simulink subsystem "EvPowertrainController2EM_r3"  (R2023a)
settings: Solver=VariableStepAuto  StartTime=0.0  StopTime=10.0  RelTol=1e-3
undefined symbols (not defined in the file): CtrlVcuAccelPdlBpts, CtrlVcuBattPnlty, CtrlVcuEMPnlty, CtrlVcuEMTrqSplitGrid, CtrlVcuEvChrgLmtBpt, CtrlVcuEvRegenBrkCutOff, CtrlVcuEvRegenBrkSpdBpt, CtrlVcuEvSocBpt, CtrlVcuFallRate, CtrlVcuMaxAccelG, CtrlVcuMaxDecelG, CtrlVcuPwrRatePnlty, CtrlVcuRiseRate, CtrlVcuRoadMuEst, CtrlVcuSftyFctr, CtrlVcuTracPwrErrPnlty, CtrlVcuTrqVecBrkThresh, CtrlVcuTrqVecMinTrq, CtrlVcuTrqVecPGain, CtrlVcuTrqVecSteerThresh, CtrlVcuTrqVecVelThresh, DriverMode, eff, EnvGrvty, PlntBrkActrBoreFrnt, PlntBrkFrntBias, PlntBrkKinFricCffFrnt, PlntBrkNumPadsFrnt, PlntBrkPadMeanRadiusFrnt, PlntBrkPrsFctr, PlntBrkRearBias, PlntDiffrntl2Eff, PlntDiffrntl2Ratio, PlntDiffrntlEff, PlntDiffrntlRatio, PlntEM1EffTbl, PlntEM1Spd, PlntEM1Trq, PlntEM1TrqEff, PlntEM2EffTbl, PlntEM2Spd, PlntEM2Trq, PlntEM2TrqEff, PlntEM3EffTbl, PlntEM3Spd, PlntEM3Trq, PlntEM3TrqEff, PlntEMWhlGearEffFL, PlntEMWhlGearEffRL, PlntEMWhlGearRatioFL, PlntEMWhlGearRatioRL, PlntTransEffSpdBpt, PlntTransEffTbl, PlntTransEffTempBpt, PlntTransEffTrqBpt, PlntTransGearNumVect, PlntTransGearRatioVect, PlntVehCGHgtAxl, PlntVehDstCGFrntAxl, PlntVehDstCGRearAxl ... (+6)
libraries: simulink x19, autolibutils x2, slpidlib x2
(part 3 of 5)

== system EvPowertrainController2EM_r3/Energy Management/Convert Whl to EMTrq Vector/4EM/Gear Eta ==
  note: Pwr >= 0, v = 1
      | Pwr < 0, v= -1
  SpdIn : Inport
  TrqIn : Inport  Port=2
  Constant : Constant  Value=PlntEMWhlGearEffFL
  Constant1 : Constant  SampleTime=-1
  Constant2 : Constant  Value=-1  SampleTime=-1
  Math Function1 : Math  Operator=pow  SignedPower=on  OutputSignalType=real
  Product1 : Product
  Switch2 : Switch  SaturateOnIntegerOverflow=off  InputSameDT=off
  eta : Outport  VectorParamsAs1DForOutWhenUnconnected=off
  wires:
  SpdIn/1 -> Product1/2
  Constant/1 -> Math Function1/1
  Constant2/1 -> Switch2/3
  Constant1/1 -> Switch2/1
  Product1/1 -> Switch2/2
  Switch2/1 -> Math Function1/2
  Math Function1/1 -> eta/1
  TrqIn/1 -> Product1/1

== system EvPowertrainController2EM_r3/Energy Management/Convert Whl to EMTrq Vector/4EM/Gear Eta1 ==
  note: Pwr >= 0, v = 1
      | Pwr < 0, v= -1
  SpdIn : Inport
  TrqIn : Inport  Port=2
  Constant : Constant  Value=PlntEMWhlGearEffRL
  Constant1 : Constant  SampleTime=-1
  Constant2 : Constant  Value=-1  SampleTime=-1
  Math Function1 : Math  Operator=pow  SignedPower=on  OutputSignalType=real
  Product1 : Product
  Switch2 : Switch  SaturateOnIntegerOverflow=off  InputSameDT=off
  eta : Outport  VectorParamsAs1DForOutWhenUnconnected=off
  wires:
  TrqIn/1 -> Product1/1
  Math Function1/1 -> eta/1
  Switch2/1 -> Math Function1/2
  Product1/1 -> Switch2/2
  Constant1/1 -> Switch2/1
  Constant2/1 -> Switch2/3
  Constant/1 -> Math Function1/1
  SpdIn/1 -> Product1/2

== system EvPowertrainController2EM_r3/Energy Management/Powertrain Constraints /Battery Constraint/Electrical Current ==
  BattV : Inport
  EMPwrElecVec : Inport  Port=2
  DC-DC Eta : Subsystem  Variant=on  VariantControlMode=label  VariantControl=Variant1  LabelModeActiveChoice=0
  Divide : Product  Inputs=*/
  Saturation : Saturate  UpperLimit=Inf  LowerLimit=0.0001
  BatteryAmp : Outport  VectorParamsAs1DForOutWhenUnconnected=off
  wires:
  Saturation/1 -> Divide/2
  BattV/1 -> Saturation/1
  Divide/1 -> BatteryAmp/1
  EMPwrElecVec/1 -> DC-DC Eta/1(In)
  DC-DC Eta/1(Out) -> Divide/1

== system EvPowertrainController2EM_r3/Energy Management/Powertrain Constraints /Battery Constraint/Power Limit Calculations ==
  note: Use Current Limits from BMS to calculate
      | discharge and charge power limits
  BattPwrDisChrgLmt : Inport
  "BattPwrChrgLmt " : Inport  Port=2
  BattV_in : Inport  Port=3
  Data Type Conversion : DataTypeConversion  SaturateOnIntegerOverflow=off  RndMeth=Floor
  Data Type Conversion1 : DataTypeConversion  SaturateOnIntegerOverflow=off  RndMeth=Floor
  Divide : Product  Inputs=*/
  Divide1 : Product  Inputs=/*
  div0protect - poly : autolibutils/div0protect - poly  thresh=.01  ZeroCross=off  ZeroCross1=on  aMode=aMode
  div0protect - poly1 : autolibutils/div0protect - poly  thresh=.01  ZeroCross=off  ZeroCross1=on  aMode=aMode
  BattCurrDischrgLmt : Outport  VectorParamsAs1DForOutWhenUnconnected=off
  BattCurrChrgLmt : Outport  Port=2  VectorParamsAs1DForOutWhenUnconnected=off
  BattPwrDischrgLmt : Outport  Port=3  VectorParamsAs1DForOutWhenUnconnected=off
  BattPwrChrgLmt : Outport  Port=4  VectorParamsAs1DForOutWhenUnconnected=off
  wires:
  div0protect - poly1/1 -> Divide/2
  div0protect - poly/1 -> Divide1/1
  Divide1/1 -> BattCurrChrgLmt/1
  BattV_in/1 -> div0protect - poly1/1, div0protect - poly/1
  Divide/1 -> BattCurrDischrgLmt/1
  Data Type Conversion1/1 -> BattPwrDischrgLmt/1
  Data Type Conversion/1 -> BattPwrChrgLmt/1
  BattPwrDisChrgLmt/1 -> Data Type Conversion1/1, Divide/1
  "BattPwrChrgLmt "/1 -> Data Type Conversion/1, Divide1/2

== system EvPowertrainController2EM_r3/Energy Management/Powertrain Constraints /EM Constraint Front/Maximum Torque ==
  note: Don't allow negative MotTrq when
      | WhlTrqCmd is >= 0
  WhlTrqCmd : Inport
  WhlEMTrqSplitVecFrnt : Inport  Port=2
  WhlTrqMaxVec : Inport  Port=3
  Compare To Zero : simulink/Logic and Bit Operations/Compare To Zero  relop=<  OutDataTypeStr=boolean
  Compare To Zero1 : simulink/Logic and Bit Operations/Compare To Zero  relop=>=  OutDataTypeStr=boolean
  Gain : Gain  Gain=-1
  Logical Operator : Logic  Operator=OR  Inputs=3  AllPortsSameDT=off  OutDataTypeStr=boolean
  Logical Operator1 : Logic  AllPortsSameDT=off  OutDataTypeStr=boolean
  Relational Operator : RelationalOperator  Operator=<  OutDataTypeStr=boolean  RndMeth=Simplest  InputSameDT=off
  Relational Operator1 : RelationalOperator  Operator=<  OutDataTypeStr=boolean  RndMeth=Simplest  InputSameDT=off
  Saturation Dynamic : simulink/Discontinuities/Saturation Dynamic  OutMin=[]  OutMax=[]  OutDataTypeStr=Inherit: Same as second input  OutDataType=fixdt(1, 16)  OutScaling=2^-10  DoSatur=off
  WhlEMTrqSatVec : Outport  VectorParamsAs1DForOutWhenUnconnected=off
  InfeasibleEMVec : Outport  Port=2  VectorParamsAs1DForOutWhenUnconnected=off
  wires:
  WhlTrqMaxVec/1 -> Saturation Dynamic/1, Relational Operator/1, Gain/1
  Logical Operator/1 -> InfeasibleEMVec/1
  Relational Operator1/1 -> Logical Operator/2
  Relational Operator/1 -> Logical Operator/1
  Saturation Dynamic/1 -> WhlEMTrqSatVec/1
  Gain/1 -> Saturation Dynamic/3, Relational Operator1/2
  WhlTrqCmd/1 -> Compare To Zero1/1
  Compare To Zero/1 -> Logical Operator1/1
  WhlEMTrqSplitVecFrnt/1 -> Compare To Zero/1, Saturation Dynamic/2, Relational Operator1/1, Relational Operator/2
  Compare To Zero1/1 -> Logical Operator1/2
  Logical Operator1/1 -> Logical Operator/3

== system EvPowertrainController2EM_r3/Energy Management/Powertrain Constraints /EM Constraint Front/Tabular Power Loss Data ==
  EMAvgSpdVec : Inport
  WhlEMTrqSatVec : Inport  Port=2
  2EM or 3EM Dual Rear : Subsystem  VariantControl=2EM or 3EM Dual Rear
  3EM Dual Front or 4EM : Subsystem  VariantControl=3EM Dual Front or 4EM
  EMPwrElecVec : Outport

== system EvPowertrainController2EM_r3/Energy Management/Powertrain Constraints /EM Constraint Front/Wheel Torque Saturation for Max g Rates ==
  WhlTrqCmd : Inport
  Tqin : Inport  Port=2
  Constant : Constant  Value=0  SampleTime=-1
  Road mu : Gain  Gain=CtrlVcuRoadMuEst
  Road mu1 : Gain  Gain=CtrlVcuRoadMuEst
  Safety Factor : Gain  Gain=CtrlVcuSftyFctr
  Safety Factor1 : Gain  Gain=CtrlVcuSftyFctr
  Saturation Dynamic3 : simulink/Discontinuities/Saturation Dynamic  OutMin=[]  OutMax=[]  OutDataTypeStr=Inherit: Same as second input  OutDataType=fixdt(1, 16)  OutScaling=2^-10  DoSatur=off
  Selector4 : Selector  InputPortWidth=2  IndexOptions=Index vector (dialog)  Indices=1  OutputSizes=1
  Selector6 : Selector  InputPortWidth=2  IndexOptions=Index vector (dialog)  Indices=1  OutputSizes=1
  Switch : Switch  Criteria=u2 > Threshold  SaturateOnIntegerOverflow=off  InputSameDT=off
  Switch1 : Switch  Criteria=u2 > Threshold  SaturateOnIntegerOverflow=off  InputSameDT=off
  Wheel Torque Limit at Max g Rates : Subsystem
  tqOut : Outport
  wires:
  WhlTrqCmd/1 -> Switch1/2, Switch/2
  Constant/1 -> Switch1/1, Switch/3
  Switch1/1 -> Saturation Dynamic3/3
  Switch/1 -> Saturation Dynamic3/1
  Safety Factor1/1 -> Switch1/3
  Safety Factor/1 -> Switch/1
  Road mu1/1 -> Safety Factor1/1
  Road mu/1 -> Safety Factor/1
  Wheel Torque Limit at Max g Rates/2(WhlTrqLmt_Brk) -> Selector6/1
  Saturation Dynamic3/1 -> tqOut/1
  Tqin/1 -> Saturation Dynamic3/2
  Selector4/1 -> Road mu/1
  Wheel Torque Limit at Max g Rates/1(WhlTrqLmt_Accel) -> Selector4/1
  Selector6/1 -> Road mu1/1

== system EvPowertrainController2EM_r3/Energy Management/Powertrain Constraints /EM Constraint Rear/Maximum Torque ==
  note: Don't allow negative MotTrq when
      | WhlTrqCmd is >= 0
  WhlTrqCmd : Inport
  WhlEMTrqSplitVecRear : Inport  Port=2
  WhlTrqMaxVec : Inport  Port=3
  Compare To Zero : simulink/Logic and Bit Operations/Compare To Zero  relop=<  OutDataTypeStr=boolean
  Compare To Zero1 : simulink/Logic and Bit Operations/Compare To Zero  relop=>=  OutDataTypeStr=boolean
  Gain : Gain  Gain=-1
  Logical Operator : Logic  Operator=OR  Inputs=3  AllPortsSameDT=off  OutDataTypeStr=boolean
  Logical Operator1 : Logic  AllPortsSameDT=off  OutDataTypeStr=boolean
  Relational Operator : RelationalOperator  Operator=<  OutDataTypeStr=boolean  RndMeth=Simplest  InputSameDT=off
  Relational Operator1 : RelationalOperator  Operator=<  OutDataTypeStr=boolean  RndMeth=Simplest  InputSameDT=off
  Saturation Dynamic : simulink/Discontinuities/Saturation Dynamic  OutMin=[]  OutMax=[]  OutDataTypeStr=Inherit: Same as second input  OutDataType=fixdt(1, 16)  OutScaling=2^-10  DoSatur=off
  WhlEMTrqSatVec : Outport  VectorParamsAs1DForOutWhenUnconnected=off
  InfeasibleEMVec : Outport  Port=2  VectorParamsAs1DForOutWhenUnconnected=off
  wires:
  Logical Operator1/1 -> Logical Operator/3
  Compare To Zero1/1 -> Logical Operator1/2
  WhlEMTrqSplitVecRear/1 -> Relational Operator/2, Relational Operator1/1, Saturation Dynamic/2, Compare To Zero/1
  Compare To Zero/1 -> Logical Operator1/1
  WhlTrqCmd/1 -> Compare To Zero1/1
  Gain/1 -> Relational Operator1/2, Saturation Dynamic/3
  Saturation Dynamic/1 -> WhlEMTrqSatVec/1
  Relational Operator/1 -> Logical Operator/1
  Relational Operator1/1 -> Logical Operator/2
  Logical Operator/1 -> InfeasibleEMVec/1
  WhlTrqMaxVec/1 -> Gain/1, Relational Operator/1, Saturation Dynamic/1

== system EvPowertrainController2EM_r3/Energy Management/Powertrain Constraints /EM Constraint Rear/Tabular Power Loss Data ==
  EMAvgSpdVec : Inport
  WhlEMTrqSatVec : Inport  Port=2
  2EM : Subsystem  VariantControl=2EM
  3EM Dual Front : Subsystem  VariantControl=3EM Dual Front
  3EM Dual Rear or 4EM : Subsystem  VariantControl=3EM Dual Rear or 4EM
  EMPwrElecVec : Outport

== system EvPowertrainController2EM_r3/Energy Management/Powertrain Constraints /EM Constraint Rear/Wheel Torque Saturation for Max g Rates ==
  WhlTrqCmd : Inport
  Tqin : Inport  Port=2
  Constant : Constant  Value=0  SampleTime=-1
  Road mu : Gain  Gain=CtrlVcuRoadMuEst
  Road mu1 : Gain  Gain=CtrlVcuRoadMuEst
  Safety Factor : Gain  Gain=CtrlVcuSftyFctr
  Safety Factor1 : Gain  Gain=CtrlVcuSftyFctr
  Saturation Dynamic3 : simulink/Discontinuities/Saturation Dynamic  OutMin=[]  OutMax=[]  OutDataTypeStr=Inherit: Same as second input  OutDataType=fixdt(1, 16)  OutScaling=2^-10  DoSatur=off
  Selector4 : Selector  InputPortWidth=2  IndexOptions=Index vector (dialog)  Indices=2  OutputSizes=1
  Selector6 : Selector  InputPortWidth=2  IndexOptions=Index vector (dialog)  Indices=2  OutputSizes=1
  Switch : Switch  Criteria=u2 > Threshold  SaturateOnIntegerOverflow=off  InputSameDT=off
  Switch1 : Switch  Criteria=u2 > Threshold  SaturateOnIntegerOverflow=off  InputSameDT=off
  Wheel Torque Limit at Max g Rates : Subsystem
  tqOut : Outport
  wires:
  WhlTrqCmd/1 -> Switch1/2, Switch/2
  Constant/1 -> Switch1/1, Switch/3
  Switch1/1 -> Saturation Dynamic3/3
  Switch/1 -> Saturation Dynamic3/1
  Safety Factor1/1 -> Switch1/3
  Safety Factor/1 -> Switch/1
  Road mu1/1 -> Safety Factor1/1
  Road mu/1 -> Safety Factor/1
  Wheel Torque Limit at Max g Rates/2(WhlTrqLmt_Brk) -> Selector6/1
  Saturation Dynamic3/1 -> tqOut/1
  Tqin/1 -> Saturation Dynamic3/2
  Selector4/1 -> Road mu/1
  Wheel Torque Limit at Max g Rates/1(WhlTrqLmt_Accel) -> Selector4/1
  Selector6/1 -> Road mu1/1

== system EvPowertrainController2EM_r3/Energy Management/Powertrain Constraints /Wheel Torque Vector Logic/Regen ==
  note: 2. If #1 is false:
      |
      | Rear Torque = Rear Torque Split Vector
  note: 2. If #1 is true:
      |
      | Rear Torque = WhlTrqCmd - WhlTrqSplitVecFront (Saturated)
  note: Check if WhlTrqCmd >= WhlTrqSplitVecFront
  note: Regen Torques are Negative
  note: Ensures rear torques never greater than
      | front torques during braking
  WhlTrqCmd : Inport
  WhlEMTrqSatVecFrnt : Inport  Port=2
  WhlEMTrqSplitVecFrnt : Inport  Port=3
  WhlEMTrqSplitVecRear : Inport  Port=4
  Action Port : ActionPort
  Add3 : Sum  Inputs=+-
  Constant1 : Constant  Value=0  SampleTime=-1
  Relational Operator : RelationalOperator  OutDataTypeStr=boolean  RndMeth=Simplest  InputSameDT=off
  Saturation Dynamic : simulink/Discontinuities/Saturation Dynamic  OutMin=[]  OutMax=[]  OutDataTypeStr=Inherit: Same as second input  OutDataType=fixdt(1, 16)  OutScaling=2^-10  DoSatur=off
  Switch1 : Switch  Criteria=u2 > Threshold  SaturateOnIntegerOverflow=off  InputSameDT=off
  WhlEMTrqSplitVecFrnt1 : Outport
  WhlEMTrqSplitVecRear1 : Outport  Port=2
  wires:
  WhlEMTrqSplitVecRear/1 -> Switch1/3
  Constant1/1 -> Saturation Dynamic/1
  Switch1/1 -> Saturation Dynamic/2
  Relational Operator/1 -> Switch1/2
  Add3/1 -> Switch1/1
  WhlEMTrqSatVecFrnt/1 -> Add3/2
  WhlTrqCmd/1 -> Relational Operator/1, Add3/1
  Saturation Dynamic/1 -> WhlEMTrqSplitVecRear1/1  "WhlEMTrqSplitVecRear"
  WhlEMTrqSplitVecFrnt/1 -> Relational Operator/2, WhlEMTrqSplitVecFrnt1/1, Saturation Dynamic/3  "WhlEMTrqSplitVecFrnt"

== system EvPowertrainController2EM_r3/Energy Management/Powertrain Constraints /Wheel Torque Vector Logic/Traction ==
  note: 2. If #1 is false:
      |
      | Front Torque = Front Torque Split Vector
  note: Check if WhlTrqCmd <= WhlTrqSplitVecRear
  note: 2. If #1 is true:
      |
      | Front Torque = WhlTrqCmd - WhlTrqSplitVecRear (Saturated)
  WhlTrqCmd : Inport
  WhlEMTrqSatVecRear : Inport  Port=2
  WhlEMTrqSplitVecFrnt : Inport  Port=3
  WhlEMTrqSplitVecRear : Inport  Port=4
  Action Port : ActionPort
  Add3 : Sum  Inputs=+-
  Relational Operator : RelationalOperator  Operator=<=  OutDataTypeStr=boolean  RndMeth=Simplest  InputSameDT=off
  Switch1 : Switch  Criteria=u2 > Threshold  SaturateOnIntegerOverflow=off  InputSameDT=off
  WhlEMTrqSplitVecFrnt1 : Outport
  WhlEMTrqSplitVecRear1 : Outport  Port=2
  wires:
  WhlEMTrqSplitVecRear/1 -> Relational Operator/2, WhlEMTrqSplitVecRear1/1  "WhlEMTrqSplitVecRear"
  Relational Operator/1 -> Switch1/2
  WhlEMTrqSplitVecFrnt/1 -> Switch1/3
  Switch1/1 -> WhlEMTrqSplitVecFrnt1/1  "WhlEMTrqSplitVecFrnt"
  WhlTrqCmd/1 -> Add3/1, Relational Operator/1
  WhlEMTrqSatVecRear/1 -> Add3/2
  Add3/1 -> Switch1/1

== system EvPowertrainController2EM_r3/Torque Vectoring/3EM/Create EMTrq Vector/3EMDualFront ==
  EMTrqSplit : Inport
  EMTrqCmd : Inport  Port=2
  Selector : Selector  InputPortWidth=3  IndexOptions=Index vector (dialog)  Indices=[3]  OutputSizes=1
  Vector Concatenate : Concatenate
  EMTrqCmdFinal : Outport
  wires:
  EMTrqSplit/1 -> Vector Concatenate/1
  Vector Concatenate/1 -> EMTrqCmdFinal/1
  EMTrqCmd/1 -> Selector/1
  Selector/1 -> Vector Concatenate/2

== system EvPowertrainController2EM_r3/Torque Vectoring/3EM/Create EMTrq Vector/3EMDualRear ==
  EMTrqSplit : Inport
  EMTrqCmd : Inport  Port=2
  Selector : Selector  InputPortWidth=3  IndexOptions=Index vector (dialog)  Indices=[1]  OutputSizes=1
  Vector Concatenate : Concatenate
  EMTrqCmdFinal : Outport
  wires:
  EMTrqCmd/1 -> Selector/1
  Vector Concatenate/1 -> EMTrqCmdFinal/1
  EMTrqSplit/1 -> Vector Concatenate/2
  Selector/1 -> Vector Concatenate/1

== system EvPowertrainController2EM_r3/Torque Vectoring/3EM/EMTrq/3EMDualFront ==
  EMSpd : Inport
  EMTrqCmd : Inport  Port=2
  1-D Lookup Table : Lookup_n-D  NumberOfTableDimensions=1  BreakpointsForDimension1=PlntEM1Spd  Table=PlntEM1Trq  ExtrapMethod=Clip  UseLastTableValue=on  InternalRulePriority=Speed  RndMeth=Simplest
  3EMDualFront : Subsystem  VariantControl=3EMDualFront
  Abs1 : Abs  SaturateOnIntegerOverflow=off
  Abs2 : Abs  SaturateOnIntegerOverflow=off
  Selector : Selector  InputPortWidth=3  IndexOptions=Index vector (dialog)  Indices=[1]  OutputSizes=1
  Selector1 : Selector  InputPortWidth=3  IndexOptions=Index vector (dialog)  Indices=[2]  OutputSizes=1
  EMTrqMax : Outport
  EMTrqL : Outport  Port=2
  EMTrqR : Outport  Port=3
  wires:
  Abs2/1 -> EMTrqMax/1
  Abs1/1 -> 1-D Lookup Table/1
  EMSpd/1 -> 3EMDualFront/1(EMSpd)
  1-D Lookup Table/1 -> Abs2/1
  3EMDualFront/1(EMSpdAvg) -> Abs1/1
  EMTrqCmd/1 -> Selector1/1, Selector/1
  Selector/1 -> EMTrqL/1
  Selector1/1 -> EMTrqR/1

== system EvPowertrainController2EM_r3/Torque Vectoring/3EM/EMTrq/3EMDualRear ==
  EMSpd : Inport
  EMTrqCmd : Inport  Port=2
  1-D Lookup Table : Lookup_n-D  NumberOfTableDimensions=1  BreakpointsForDimension1=PlntEM3Spd  Table=PlntEM3Trq  ExtrapMethod=Clip  UseLastTableValue=on  InternalRulePriority=Speed  RndMeth=Simplest
  3EMDualRear : Subsystem  VariantControl=3EMDualRear
  Abs1 : Abs  SaturateOnIntegerOverflow=off
  Abs2 : Abs  SaturateOnIntegerOverflow=off
  Selector : Selector  InputPortWidth=3  IndexOptions=Index vector (dialog)  Indices=[2]  OutputSizes=1
  Selector1 : Selector  InputPortWidth=3  IndexOptions=Index vector (dialog)  Indices=[3]  OutputSizes=1
  EMTrqMax : Outport
  EMTrqL : Outport  Port=2
  EMTrqR : Outport  Port=3
  wires:
  Abs2/1 -> EMTrqMax/1
  3EMDualRear/1(EMSpdAvg) -> Abs1/1
  1-D Lookup Table/1 -> Abs2/1
  EMSpd/1 -> 3EMDualRear/1(EMSpd)
  Abs1/1 -> 1-D Lookup Table/1
  Selector1/1 -> EMTrqR/1
  Selector/1 -> EMTrqL/1
  EMTrqCmd/1 -> Selector1/1, Selector/1

== system EvPowertrainController2EM_r3/Torque Vectoring/4EM/EMTrq/Dual Front ==
  EMSpd : Inport
  EMTrqCmd : Inport  Port=2
  1-D Lookup Table : Lookup_n-D  NumberOfTableDimensions=1  BreakpointsForDimension1=PlntEM1Spd  Table=PlntEM1Trq  ExtrapMethod=Clip  UseLastTableValue=on  InternalRulePriority=Speed  RndMeth=Simplest
  3EMDualFrnt : Subsystem  VariantControl=3EMDualFront
  Abs1 : Abs  SaturateOnIntegerOverflow=off
  Abs2 : Abs  SaturateOnIntegerOverflow=off
  Selector : Selector  InputPortWidth=4  IndexOptions=Index vector (dialog)  Indices=[1]  OutputSizes=1
  Selector1 : Selector  InputPortWidth=4  IndexOptions=Index vector (dialog)  Indices=[2]  OutputSizes=1
  EMTrqMaxFrnt : Outport
  EMTrqFL : Outport  Port=2
  EMTrqFR : Outport  Port=3
  wires:
  Abs2/1 -> EMTrqMaxFrnt/1
  Selector1/1 -> EMTrqFR/1
  Selector/1 -> EMTrqFL/1
  EMTrqCmd/1 -> Selector/1, Selector1/1
  3EMDualFrnt/1(EMSpdAvg) -> Abs1/1
  1-D Lookup Table/1 -> Abs2/1
  EMSpd/1 -> 3EMDualFrnt/1(EMSpd)
  Abs1/1 -> 1-D Lookup Table/1

== system EvPowertrainController2EM_r3/Torque Vectoring/4EM/EMTrq/Dual Rear ==
  EMSpd : Inport
  EMTrqCmd : Inport  Port=2
  1-D Lookup Table : Lookup_n-D  NumberOfTableDimensions=1  BreakpointsForDimension1=PlntEM3Spd  Table=PlntEM3Trq  ExtrapMethod=Clip  UseLastTableValue=on  InternalRulePriority=Speed  RndMeth=Simplest
  3EMDualRear : Subsystem  VariantControl=3EMDualRear
  Abs1 : Abs  SaturateOnIntegerOverflow=off
  Abs2 : Abs  SaturateOnIntegerOverflow=off
  Selector : Selector  InputPortWidth=4  IndexOptions=Index vector (dialog)  Indices=[3]  OutputSizes=1
  Selector1 : Selector  InputPortWidth=4  IndexOptions=Index vector (dialog)  Indices=[4]  OutputSizes=1
  EMTrqMaxRear : Outport
  EMTrqRL : Outport  Port=2
  EMTrqRR : Outport  Port=3
  wires:
  Abs2/1 -> EMTrqMaxRear/1
  EMTrqCmd/1 -> Selector/1, Selector1/1
  Selector/1 -> EMTrqRL/1
  Selector1/1 -> EMTrqRR/1
  Abs1/1 -> 1-D Lookup Table/1
  EMSpd/1 -> 3EMDualRear/1(EMSpd)
  1-D Lookup Table/1 -> Abs2/1
  3EMDualRear/1(EMSpdAvg) -> Abs1/1

== system EvPowertrainController2EM_r3/Accel Pedal to Traction Wheel Torque Request/EM2WhlTrq/2EM/EMTrq2WhlTrqFrnt/No Transmission ==
  EMTrqCmd : Inport
  EMSpd : Inport  Port=2
  Diff Eta : Subsystem
  Divide2 : Product  Inputs=**
  Gain3 : Gain  Gain=PlntDiffrntlRatio
  WhlMotTrq : Outport  VectorParamsAs1DForOutWhenUnconnected=off
  wires:
  Gain3/1 -> Divide2/2
  Divide2/1 -> WhlMotTrq/1
  EMSpd/1 -> Diff Eta/1(SpdIn)
  EMTrqCmd/1 -> Diff Eta/2(TrqIn), Gain3/1
  Diff Eta/1(eta) -> Divide2/1

== system EvPowertrainController2EM_r3/Accel Pedal to Traction Wheel Torque Request/EM2WhlTrq/2EM/EMTrq2WhlTrqFrnt/Transmission ==
  Gear : Inport
  EMTrqCmd : Inport  Port=2
  EMSpd : Inport  Port=3
  Diff Eta : Subsystem
  Divide : Product  Inputs=**
  Divide1 : Product  Inputs=**
  Divide2 : Product  Inputs=**
  Divide3 : Product  Inputs=*/
  Gain : Gain  Gain=PlntDiffrntlRatio
  Gear ratio look up : LookupNDDirect  NumberOfTableDimensions=1  Table=PlntTransGearRatioVect
  Trans Eta : Subsystem
  WhlMotTrq : Outport  VectorParamsAs1DForOutWhenUnconnected=off
  wires:
  EMSpd/1 -> Trans Eta/2(SpdIn), [Spd]
  EMTrqCmd/1 -> Trans Eta/1(TrqIn), Divide/2
  Divide3/1 -> Diff Eta/1(SpdIn)
  [Spd] -> Divide3/1
  Diff Eta/1(eta) -> Divide2/1
  Divide2/1 -> WhlMotTrq/1
  Divide1/1 -> Gain/1, Diff Eta/2(TrqIn)
  Trans Eta/1(eta) -> Divide1/1
  Gear/1 -> Gear ratio look up/1, Trans Eta/3(Gear)
  Divide/1 -> Divide1/2
  Gear ratio look up/1 -> Divide/1, Divide3/2
  Gain/1 -> Divide2/2

== system EvPowertrainController2EM_r3/Accel Pedal to Traction Wheel Torque Request/EM2WhlTrq/2EM/EMTrq2WhlTrqRear/No Transmission ==
  EMTrqCmd : Inport
  EMSpd : Inport  Port=2
  Diff Eta : Subsystem
  Divide2 : Product  Inputs=**
  Gain3 : Gain  Gain=PlntDiffrntl2Ratio
  WhlMotTrq : Outport  VectorParamsAs1DForOutWhenUnconnected=off
  wires:
  Gain3/1 -> Divide2/2
  Divide2/1 -> WhlMotTrq/1
  EMSpd/1 -> Diff Eta/1(SpdIn)
  EMTrqCmd/1 -> Diff Eta/2(TrqIn), Gain3/1
  Diff Eta/1(eta) -> Divide2/1

== system EvPowertrainController2EM_r3/Accel Pedal to Traction Wheel Torque Request/EM2WhlTrq/2EM/EMTrq2WhlTrqRear/Transmission ==
  Gear : Inport
  EMTrqCmd : Inport  Port=2
  EMSpd : Inport  Port=3
  Diff Eta : Subsystem
  Divide : Product  Inputs=**
  Divide1 : Product  Inputs=**
  Divide2 : Product  Inputs=**
  Divide3 : Product  Inputs=*/
  Gain : Gain  Gain=PlntDiffrntl2Ratio
  Gear ratio look up : LookupNDDirect  NumberOfTableDimensions=1  Table=PlntTransGearRatioVect
  Trans Eta : Subsystem
  WhlMotTrq : Outport  VectorParamsAs1DForOutWhenUnconnected=off
  wires:
  Gain/1 -> Divide2/2
  Gear ratio look up/1 -> Divide3/2, Divide/1
  Divide/1 -> Divide1/2
  Gear/1 -> Trans Eta/3(Gear), Gear ratio look up/1
  Trans Eta/1(eta) -> Divide1/1
  Divide1/1 -> Diff Eta/2(TrqIn), Gain/1
  Divide2/1 -> WhlMotTrq/1
  Diff Eta/1(eta) -> Divide2/1
  [Spd] -> Divide3/1
  Divide3/1 -> Diff Eta/1(SpdIn)
  EMTrqCmd/1 -> Divide/2, Trans Eta/1(TrqIn)
  EMSpd/1 -> [Spd], Trans Eta/2(SpdIn)

== system EvPowertrainController2EM_r3/Accel Pedal to Traction Wheel Torque Request/EM2WhlTrq/2EM/VehSpd2EMSpd/No Transmission ==
  VehSpd : Inport
  Gain1 : Gain  Gain=PlntDiffrntlRatio
  Gain2 : Gain  Gain=PlntDiffrntl2Ratio
  Gain3 : Gain  Gain=1 / PlntWhlLdRadius
  EMSpdFrntAxl : Outport  VectorParamsAs1DForOutWhenUnconnected=off
  EMSpdRearAxl : Outport  Port=2  VectorParamsAs1DForOutWhenUnconnected=off
  wires:
  Gain2/1 -> EMSpdRearAxl/1
  Gain3/1 -> Gain2/1, Gain1/1
  Gain1/1 -> EMSpdFrntAxl/1
  VehSpd/1 -> Gain3/1

== system EvPowertrainController2EM_r3/Accel Pedal to Traction Wheel Torque Request/EM2WhlTrq/2EM/VehSpd2EMSpd/Transmission ==
  Gear : Inport
  VehSpd : Inport  Port=2
  Divide1 : Product  Inputs=**
  Gain1 : Gain  Gain=PlntDiffrntlRatio
  Gain2 : Gain  Gain=PlntDiffrntl2Ratio
  Gain3 : Gain  Gain=1 / PlntWhlLdRadius
  Gear ratio look up : LookupNDDirect  NumberOfTableDimensions=1  Table=PlntTransGearRatioVect
  EMSpdFrntAxl : Outport  VectorParamsAs1DForOutWhenUnconnected=off
  EMSpdRearAxl : Outport  Port=2  VectorParamsAs1DForOutWhenUnconnected=off
  wires:
  Divide1/1 -> EMSpdRearAxl/1
  Gain2/1 -> Divide1/2
  Gear ratio look up/1 -> Divide1/1
  Gain1/1 -> EMSpdFrntAxl/1
  Gain3/1 -> Gain1/1, Gain2/1
  Gear/1 -> Gear ratio look up/1
  VehSpd/1 -> Gain3/1

== system EvPowertrainController2EM_r3/Accel Pedal to Traction Wheel Torque Request/EM2WhlTrq/3EM Dual Front/EMTrq2WhlTrqFrnt/No Transmission ==
  EMTrqCmd : Inport
  EMSpd : Inport  Port=2
  Divide2 : Product  Inputs=**
  Dual EMs : Gain  Gain=2
  Gain3 : Gain  Gain=PlntEMWhlGearRatioFL
  Gear Eta : Subsystem
  WhlMotTrq : Outport  VectorParamsAs1DForOutWhenUnconnected=off
  wires:
  Dual EMs/1 -> Gain3/1, Gear Eta/2(TrqIn)
  Gear Eta/1(eta) -> Divide2/1
  EMTrqCmd/1 -> Dual EMs/1
  EMSpd/1 -> Gear Eta/1(SpdIn)
  Divide2/1 -> WhlMotTrq/1
  Gain3/1 -> Divide2/2

== system EvPowertrainController2EM_r3/Accel Pedal to Traction Wheel Torque Request/EM2WhlTrq/3EM Dual Front/EMTrq2WhlTrqFrnt/Transmission ==
  Gear : Inport
  EMTrqCmd : Inport  Port=2
  EMSpd : Inport  Port=3
  Diff Eta : Subsystem
  Divide : Product  Inputs=**
  Divide1 : Product  Inputs=**
  Divide2 : Product  Inputs=**
  Divide3 : Product  Inputs=*/
  Gain : Gain  Gain=PlntDiffrntlRatio
  Gear ratio look up : LookupNDDirect  NumberOfTableDimensions=1  Table=PlntTransGearRatioVect
  Trans Eta : Subsystem
  WhlMotTrq : Outport  VectorParamsAs1DForOutWhenUnconnected=off
  wires:
  Gain/1 -> Divide2/2
  Gear ratio look up/1 -> Divide3/2, Divide/1
  Divide/1 -> Divide1/2
  Gear/1 -> Trans Eta/3(Gear), Gear ratio look up/1
  Trans Eta/1(eta) -> Divide1/1
  Divide1/1 -> Diff Eta/2(TrqIn), Gain/1
  Divide2/1 -> WhlMotTrq/1
  Diff Eta/1(eta) -> Divide2/1
  [Spd] -> Divide3/1
  Divide3/1 -> Diff Eta/1(SpdIn)
  EMTrqCmd/1 -> Divide/2, Trans Eta/1(TrqIn)
  EMSpd/1 -> [Spd], Trans Eta/2(SpdIn)

== system EvPowertrainController2EM_r3/Accel Pedal to Traction Wheel Torque Request/EM2WhlTrq/3EM Dual Front/EMTrq2WhlTrqRear/No Transmission ==
  EMTrqCmd : Inport
  EMSpd : Inport  Port=2
  Diff Eta : Subsystem
  Divide2 : Product  Inputs=**
  Gain3 : Gain  Gain=PlntDiffrntl2Ratio
  WhlMotTrq : Outport  VectorParamsAs1DForOutWhenUnconnected=off
  wires:
  Diff Eta/1(eta) -> Divide2/1
  EMTrqCmd/1 -> Gain3/1, Diff Eta/2(TrqIn)
  EMSpd/1 -> Diff Eta/1(SpdIn)
  Divide2/1 -> WhlMotTrq/1
  Gain3/1 -> Divide2/2

== system EvPowertrainController2EM_r3/Accel Pedal to Traction Wheel Torque Request/EM2WhlTrq/3EM Dual Front/EMTrq2WhlTrqRear/Transmission ==
  Gear : Inport
  EMTrqCmd : Inport  Port=2
  EMSpd : Inport  Port=3
  Diff Eta : Subsystem
  Divide : Product  Inputs=**
  Divide1 : Product  Inputs=**
  Divide2 : Product  Inputs=**
  Divide3 : Product  Inputs=*/
  Gain : Gain  Gain=PlntDiffrntl2Ratio
  Gear ratio look up : LookupNDDirect  NumberOfTableDimensions=1  Table=PlntTransGearRatioVect
  Trans Eta : Subsystem
  WhlMotTrq : Outport  VectorParamsAs1DForOutWhenUnconnected=off
  wires:
  EMSpd/1 -> Trans Eta/2(SpdIn), [Spd]
  EMTrqCmd/1 -> Trans Eta/1(TrqIn), Divide/2
  Divide3/1 -> Diff Eta/1(SpdIn)
  [Spd] -> Divide3/1
  Diff Eta/1(eta) -> Divide2/1
  Divide2/1 -> WhlMotTrq/1
  Divide1/1 -> Gain/1, Diff Eta/2(TrqIn)
  Trans Eta/1(eta) -> Divide1/1
  Gear/1 -> Gear ratio look up/1, Trans Eta/3(Gear)
  Divide/1 -> Divide1/2
  Gear ratio look up/1 -> Divide/1, Divide3/2
  Gain/1 -> Divide2/2

== system EvPowertrainController2EM_r3/Accel Pedal to Traction Wheel Torque Request/EM2WhlTrq/3EM Dual Front/VehSpd2EMSpd/No Transmission ==
  VehSpd : Inport
  Gain1 : Gain  Gain=PlntEMWhlGearRatioFL
  Gain2 : Gain  Gain=PlntDiffrntl2Ratio
  Gain3 : Gain  Gain=1 / PlntWhlLdRadius
  EMSpdFrntAxl : Outport  VectorParamsAs1DForOutWhenUnconnected=off
  EMSpdRearAxl : Outport  Port=2  VectorParamsAs1DForOutWhenUnconnected=off
  wires:
  VehSpd/1 -> Gain3/1
  Gain1/1 -> EMSpdFrntAxl/1
  Gain3/1 -> Gain1/1, Gain2/1
  Gain2/1 -> EMSpdRearAxl/1

== system EvPowertrainController2EM_r3/Accel Pedal to Traction Wheel Torque Request/EM2WhlTrq/3EM Dual Front/VehSpd2EMSpd/Transmission ==
  Gear : Inport
  VehSpd : Inport  Port=2
  Divide1 : Product  Inputs=**
  Gain1 : Gain  Gain=PlntDiffrntlRatio
  Gain2 : Gain  Gain=PlntDiffrntl2Ratio
  Gain3 : Gain  Gain=1 / PlntWhlLdRadius
  Gear ratio look up : LookupNDDirect  NumberOfTableDimensions=1  Table=PlntTransGearRatioVect
  EMSpdFrntAxl : Outport  VectorParamsAs1DForOutWhenUnconnected=off
  EMSpdRearAxl : Outport  Port=2  VectorParamsAs1DForOutWhenUnconnected=off
  wires:
  VehSpd/1 -> Gain3/1
  Gear/1 -> Gear ratio look up/1
  Gain3/1 -> Gain2/1, Gain1/1
  Gain1/1 -> EMSpdFrntAxl/1
  Gear ratio look up/1 -> Divide1/1
  Gain2/1 -> Divide1/2
  Divide1/1 -> EMSpdRearAxl/1

== system EvPowertrainController2EM_r3/Accel Pedal to Traction Wheel Torque Request/EM2WhlTrq/3EM Dual Rear/EMTrq2WhlTrqFrnt/No Transmission ==
  EMTrqCmd : Inport
  EMSpd : Inport  Port=2
  Diff Eta : Subsystem
  Divide2 : Product  Inputs=**
  Gain3 : Gain  Gain=PlntDiffrntlRatio
  WhlMotTrq : Outport  VectorParamsAs1DForOutWhenUnconnected=off
  wires:
  Gain3/1 -> Divide2/2
  Divide2/1 -> WhlMotTrq/1
  EMSpd/1 -> Diff Eta/1(SpdIn)
  EMTrqCmd/1 -> Diff Eta/2(TrqIn), Gain3/1
  Diff Eta/1(eta) -> Divide2/1

== system EvPowertrainController2EM_r3/Accel Pedal to Traction Wheel Torque Request/EM2WhlTrq/3EM Dual Rear/EMTrq2WhlTrqFrnt/Transmission ==
  Gear : Inport
  EMTrqCmd : Inport  Port=2
  EMSpd : Inport  Port=3
  Diff Eta : Subsystem
  Divide : Product  Inputs=**
  Divide1 : Product  Inputs=**
  Divide2 : Product  Inputs=**
  Divide3 : Product  Inputs=*/
  Gain : Gain  Gain=PlntDiffrntlRatio
  Gear ratio look up : LookupNDDirect  NumberOfTableDimensions=1  Table=PlntTransGearRatioVect
  Trans Eta : Subsystem
  WhlMotTrq : Outport  VectorParamsAs1DForOutWhenUnconnected=off
  wires:
  EMSpd/1 -> Trans Eta/2(SpdIn), [Spd]
  EMTrqCmd/1 -> Trans Eta/1(TrqIn), Divide/2
  Divide3/1 -> Diff Eta/1(SpdIn)
  [Spd] -> Divide3/1
  Diff Eta/1(eta) -> Divide2/1
  Divide2/1 -> WhlMotTrq/1
  Divide1/1 -> Gain/1, Diff Eta/2(TrqIn)
  Trans Eta/1(eta) -> Divide1/1
  Gear/1 -> Gear ratio look up/1, Trans Eta/3(Gear)
  Divide/1 -> Divide1/2
  Gear ratio look up/1 -> Divide/1, Divide3/2
  Gain/1 -> Divide2/2

== system EvPowertrainController2EM_r3/Accel Pedal to Traction Wheel Torque Request/EM2WhlTrq/3EM Dual Rear/EMTrq2WhlTrqRear/No Transmission ==
  EMTrqCmd : Inport
  EMSpd : Inport  Port=2
  Divide2 : Product  Inputs=**
  Dual EMs : Gain  Gain=2
  Gain3 : Gain  Gain=PlntEMWhlGearRatioRL
  Gear Eta : Subsystem
  WhlMotTrq : Outport  VectorParamsAs1DForOutWhenUnconnected=off
  wires:
  Dual EMs/1 -> Gear Eta/2(TrqIn), Gain3/1
  Gain3/1 -> Divide2/2
  Divide2/1 -> WhlMotTrq/1
  EMSpd/1 -> Gear Eta/1(SpdIn)
  EMTrqCmd/1 -> Dual EMs/1
  Gear Eta/1(eta) -> Divide2/1

== system EvPowertrainController2EM_r3/Accel Pedal to Traction Wheel Torque Request/EM2WhlTrq/3EM Dual Rear/EMTrq2WhlTrqRear/Transmission ==
  Gear : Inport
  EMTrqCmd : Inport  Port=2
  EMSpd : Inport  Port=3
  Diff Eta : Subsystem
  Divide : Product  Inputs=**
  Divide1 : Product  Inputs=**
  Divide2 : Product  Inputs=**
  Divide3 : Product  Inputs=*/
  Gain : Gain  Gain=PlntDiffrntl2Ratio
  Gear ratio look up : LookupNDDirect  NumberOfTableDimensions=1  Table=PlntTransGearRatioVect
  Trans Eta : Subsystem
  WhlMotTrq : Outport  VectorParamsAs1DForOutWhenUnconnected=off
  wires:
  Gain/1 -> Divide2/2
  Gear ratio look up/1 -> Divide3/2, Divide/1
  Divide/1 -> Divide1/2
  Gear/1 -> Trans Eta/3(Gear), Gear ratio look up/1
  Trans Eta/1(eta) -> Divide1/1
  Divide1/1 -> Diff Eta/2(TrqIn), Gain/1
  Divide2/1 -> WhlMotTrq/1
  Diff Eta/1(eta) -> Divide2/1
  [Spd] -> Divide3/1
  Divide3/1 -> Diff Eta/1(SpdIn)
  EMTrqCmd/1 -> Divide/2, Trans Eta/1(TrqIn)
  EMSpd/1 -> [Spd], Trans Eta/2(SpdIn)

== system EvPowertrainController2EM_r3/Accel Pedal to Traction Wheel Torque Request/EM2WhlTrq/3EM Dual Rear/VehSpd2EMSpd/No Transmission ==
  VehSpd : Inport
  Gain1 : Gain  Gain=PlntDiffrntlRatio
  Gain2 : Gain  Gain=PlntEMWhlGearRatioRL
  Gain3 : Gain  Gain=1 / PlntWhlLdRadius
  EMSpdFrntAxl : Outport  VectorParamsAs1DForOutWhenUnconnected=off
  EMSpdRearAxl : Outport  Port=2  VectorParamsAs1DForOutWhenUnconnected=off
  wires:
  Gain2/1 -> EMSpdRearAxl/1
  Gain3/1 -> Gain2/1, Gain1/1
  Gain1/1 -> EMSpdFrntAxl/1
  VehSpd/1 -> Gain3/1

== system EvPowertrainController2EM_r3/Accel Pedal to Traction Wheel Torque Request/EM2WhlTrq/3EM Dual Rear/VehSpd2EMSpd/Transmission ==
  Gear : Inport
  VehSpd : Inport  Port=2
  Divide1 : Product  Inputs=**
  Gain1 : Gain  Gain=PlntDiffrntlRatio
  Gain2 : Gain  Gain=PlntDiffrntl2Ratio
  Gain3 : Gain  Gain=1 / PlntWhlLdRadius
  Gear ratio look up : LookupNDDirect  NumberOfTableDimensions=1  Table=PlntTransGearRatioVect
  EMSpdFrntAxl : Outport  VectorParamsAs1DForOutWhenUnconnected=off
  EMSpdRearAxl : Outport  Port=2  VectorParamsAs1DForOutWhenUnconnected=off
  wires:
  Divide1/1 -> EMSpdRearAxl/1
  Gain2/1 -> Divide1/2
  Gear ratio look up/1 -> Divide1/1
  Gain1/1 -> EMSpdFrntAxl/1
  Gain3/1 -> Gain1/1, Gain2/1
  Gear/1 -> Gear ratio look up/1
  VehSpd/1 -> Gain3/1

== system EvPowertrainController2EM_r3/Accel Pedal to Traction Wheel Torque Request/EM2WhlTrq/4EM/EMTrq2WhlTrqFrnt/No Transmission ==
  EMTrqCmd : Inport
  EMSpd : Inport  Port=2
  Divide2 : Product  Inputs=**
  Dual EMs : Gain  Gain=2
  Gain3 : Gain  Gain=PlntEMWhlGearRatioFL
  Gear Eta : Subsystem
  WhlMotTrq : Outport  VectorParamsAs1DForOutWhenUnconnected=off
  wires:
  Dual EMs/1 -> Gain3/1, Gear Eta/2(TrqIn)
  Gear Eta/1(eta) -> Divide2/1
  EMTrqCmd/1 -> Dual EMs/1
  EMSpd/1 -> Gear Eta/1(SpdIn)
  Divide2/1 -> WhlMotTrq/1
  Gain3/1 -> Divide2/2

== system EvPowertrainController2EM_r3/Accel Pedal to Traction Wheel Torque Request/EM2WhlTrq/4EM/EMTrq2WhlTrqFrnt/Transmission ==
  Gear : Inport
  EMTrqCmd : Inport  Port=2
  EMSpd : Inport  Port=3
  Diff Eta : Subsystem
  Divide : Product  Inputs=**
  Divide1 : Product  Inputs=**
  Divide2 : Product  Inputs=**
  Divide3 : Product  Inputs=*/
  Gain : Gain  Gain=PlntDiffrntlRatio
  Gear ratio look up : LookupNDDirect  NumberOfTableDimensions=1  Table=PlntTransGearRatioVect
  Trans Eta : Subsystem
  WhlMotTrq : Outport  VectorParamsAs1DForOutWhenUnconnected=off
  wires:
  Gain/1 -> Divide2/2
  Gear ratio look up/1 -> Divide3/2, Divide/1
  Divide/1 -> Divide1/2
  Gear/1 -> Trans Eta/3(Gear), Gear ratio look up/1
  Trans Eta/1(eta) -> Divide1/1
  Divide1/1 -> Diff Eta/2(TrqIn), Gain/1
  Divide2/1 -> WhlMotTrq/1
  Diff Eta/1(eta) -> Divide2/1
  [Spd] -> Divide3/1
  Divide3/1 -> Diff Eta/1(SpdIn)
  EMTrqCmd/1 -> Divide/2, Trans Eta/1(TrqIn)
  EMSpd/1 -> [Spd], Trans Eta/2(SpdIn)

== system EvPowertrainController2EM_r3/Accel Pedal to Traction Wheel Torque Request/EM2WhlTrq/4EM/EMTrq2WhlTrqRear/No Transmission ==
  EMTrqCmd : Inport
  EMSpd : Inport  Port=2
  Divide2 : Product  Inputs=**
  Dual EMs : Gain  Gain=2
  Gain3 : Gain  Gain=PlntEMWhlGearRatioRL
  Gear Eta : Subsystem
  WhlMotTrq : Outport  VectorParamsAs1DForOutWhenUnconnected=off
  wires:
  Dual EMs/1 -> Gain3/1, Gear Eta/2(TrqIn)
  Gear Eta/1(eta) -> Divide2/1
  EMTrqCmd/1 -> Dual EMs/1
  EMSpd/1 -> Gear Eta/1(SpdIn)
  Divide2/1 -> WhlMotTrq/1
  Gain3/1 -> Divide2/2

== system EvPowertrainController2EM_r3/Accel Pedal to Traction Wheel Torque Request/EM2WhlTrq/4EM/EMTrq2WhlTrqRear/Transmission ==
  Gear : Inport
  EMTrqCmd : Inport  Port=2
  EMSpd : Inport  Port=3
  Diff Eta : Subsystem
  Divide : Product  Inputs=**
  Divide1 : Product  Inputs=**
  Divide2 : Product  Inputs=**
  Divide3 : Product  Inputs=*/
  Gain : Gain  Gain=PlntDiffrntl2Ratio
  Gear ratio look up : LookupNDDirect  NumberOfTableDimensions=1  Table=PlntTransGearRatioVect
  Trans Eta : Subsystem
  WhlMotTrq : Outport  VectorParamsAs1DForOutWhenUnconnected=off
  wires:
  EMSpd/1 -> Trans Eta/2(SpdIn), [Spd]
  EMTrqCmd/1 -> Trans Eta/1(TrqIn), Divide/2
  Divide3/1 -> Diff Eta/1(SpdIn)
  [Spd] -> Divide3/1
  Diff Eta/1(eta) -> Divide2/1
  Divide2/1 -> WhlMotTrq/1
  Divide1/1 -> Gain/1, Diff Eta/2(TrqIn)
  Trans Eta/1(eta) -> Divide1/1
  Gear/1 -> Gear ratio look up/1, Trans Eta/3(Gear)
  Divide/1 -> Divide1/2
  Gear ratio look up/1 -> Divide/1, Divide3/2
  Gain/1 -> Divide2/2

== system EvPowertrainController2EM_r3/Accel Pedal to Traction Wheel Torque Request/EM2WhlTrq/4EM/VehSpd2EMSpd/No Transmission ==
  VehSpd : Inport
  Gain1 : Gain  Gain=PlntEMWhlGearRatioFL
  Gain2 : Gain  Gain=PlntEMWhlGearRatioRL
  Gain3 : Gain  Gain=1 / PlntWhlLdRadius
  EMSpdFrntAxl : Outport  VectorParamsAs1DForOutWhenUnconnected=off
  EMSpdRearAxl : Outport  Port=2  VectorParamsAs1DForOutWhenUnconnected=off
  wires:
  VehSpd/1 -> Gain3/1
  Gain1/1 -> EMSpdFrntAxl/1
  Gain3/1 -> Gain2/1, Gain1/1
  Gain2/1 -> EMSpdRearAxl/1

== system EvPowertrainController2EM_r3/Accel Pedal to Traction Wheel Torque Request/EM2WhlTrq/4EM/VehSpd2EMSpd/Transmission ==
  Gear : Inport
  VehSpd : Inport  Port=2
  Divide1 : Product  Inputs=**
  Gain1 : Gain  Gain=PlntDiffrntlRatio
  Gain2 : Gain  Gain=PlntDiffrntl2Ratio
  Gain3 : Gain  Gain=1 / PlntWhlLdRadius
  Gear ratio look up : LookupNDDirect  NumberOfTableDimensions=1  Table=PlntTransGearRatioVect
  EMSpdFrntAxl : Outport  VectorParamsAs1DForOutWhenUnconnected=off
  EMSpdRearAxl : Outport  Port=2  VectorParamsAs1DForOutWhenUnconnected=off
  wires:
  VehSpd/1 -> Gain3/1
  Gear/1 -> Gear ratio look up/1
  Gain3/1 -> Gain2/1, Gain1/1
  Gain1/1 -> EMSpdFrntAxl/1
  Gear ratio look up/1 -> Divide1/1
  Gain2/1 -> Divide1/2
  Divide1/1 -> EMSpdRearAxl/1

== system EvPowertrainController2EM_r3/Energy Management/Calculate Average EMSpd and Wheel Torque Curves for Front and Rear Axles/2EM/EMTrq2WhlTrqFrnt/No Transmission ==
  EMTrqCmd : Inport
  EMSpd : Inport  Port=2
  Diff Eta : Subsystem
  Divide2 : Product  Inputs=**
  Gain3 : Gain  Gain=PlntDiffrntlRatio
  WhlMotTrq : Outport  VectorParamsAs1DForOutWhenUnconnected=off
  wires:
  Gain3/1 -> Divide2/2
  Divide2/1 -> WhlMotTrq/1
  EMSpd/1 -> Diff Eta/1(SpdIn)
  EMTrqCmd/1 -> Diff Eta/2(TrqIn), Gain3/1
  Diff Eta/1(eta) -> Divide2/1

== system EvPowertrainController2EM_r3/Energy Management/Calculate Average EMSpd and Wheel Torque Curves for Front and Rear Axles/2EM/EMTrq2WhlTrqFrnt/Transmission ==
  Gear : Inport
  EMTrqCmd : Inport  Port=2
  EMSpd : Inport  Port=3
  Diff Eta : Subsystem
  Divide : Product  Inputs=**
  Divide1 : Product  Inputs=**
  Divide2 : Product  Inputs=**
  Divide3 : Product  Inputs=*/
  Gain : Gain  Gain=PlntDiffrntlRatio
  Gear ratio look up : LookupNDDirect  NumberOfTableDimensions=1  Table=PlntTransGearRatioVect
  Trans Eta : Subsystem
  WhlMotTrq : Outport  VectorParamsAs1DForOutWhenUnconnected=off
  wires:
  EMSpd/1 -> Trans Eta/2(SpdIn), [Spd]
  EMTrqCmd/1 -> Trans Eta/1(TrqIn), Divide/2
  Divide3/1 -> Diff Eta/1(SpdIn)
  [Spd] -> Divide3/1
  Diff Eta/1(eta) -> Divide2/1
  Divide2/1 -> WhlMotTrq/1
  Divide1/1 -> Gain/1, Diff Eta/2(TrqIn)
  Trans Eta/1(eta) -> Divide1/1
  Gear/1 -> Gear ratio look up/1, Trans Eta/3(Gear)
  Divide/1 -> Divide1/2
  Gear ratio look up/1 -> Divide/1, Divide3/2
  Gain/1 -> Divide2/2

== system EvPowertrainController2EM_r3/Energy Management/Calculate Average EMSpd and Wheel Torque Curves for Front and Rear Axles/2EM/EMTrq2WhlTrqRear/No Transmission ==
  EMTrqCmd : Inport
  EMSpd : Inport  Port=2
  Diff Eta : Subsystem
  Divide2 : Product  Inputs=**
  Gain3 : Gain  Gain=PlntDiffrntl2Ratio
  WhlMotTrq : Outport  VectorParamsAs1DForOutWhenUnconnected=off
  wires:
  Gain3/1 -> Divide2/2
  Divide2/1 -> WhlMotTrq/1
  EMSpd/1 -> Diff Eta/1(SpdIn)
  EMTrqCmd/1 -> Diff Eta/2(TrqIn), Gain3/1
  Diff Eta/1(eta) -> Divide2/1

== system EvPowertrainController2EM_r3/Energy Management/Calculate Average EMSpd and Wheel Torque Curves for Front and Rear Axles/2EM/EMTrq2WhlTrqRear/Transmission ==
  Gear : Inport
  EMTrqCmd : Inport  Port=2
  EMSpd : Inport  Port=3
  Diff Eta : Subsystem
  Divide : Product  Inputs=**
  Divide1 : Product  Inputs=**
  Divide2 : Product  Inputs=**
  Divide3 : Product  Inputs=*/
  Gain : Gain  Gain=PlntDiffrntl2Ratio
  Gear ratio look up : LookupNDDirect  NumberOfTableDimensions=1  Table=PlntTransGearRatioVect
  Trans Eta : Subsystem
  WhlMotTrq : Outport  VectorParamsAs1DForOutWhenUnconnected=off
  wires:
  Gain/1 -> Divide2/2
  Gear ratio look up/1 -> Divide3/2, Divide/1
  Divide/1 -> Divide1/2
  Gear/1 -> Trans Eta/3(Gear), Gear ratio look up/1
  Trans Eta/1(eta) -> Divide1/1
  Divide1/1 -> Diff Eta/2(TrqIn), Gain/1
  Divide2/1 -> WhlMotTrq/1
  Diff Eta/1(eta) -> Divide2/1
  [Spd] -> Divide3/1
  Divide3/1 -> Diff Eta/1(SpdIn)
  EMTrqCmd/1 -> Divide/2, Trans Eta/1(TrqIn)
  EMSpd/1 -> [Spd], Trans Eta/2(SpdIn)

== system EvPowertrainController2EM_r3/Energy Management/Calculate Average EMSpd and Wheel Torque Curves for Front and Rear Axles/3EM Dual Front/EMTrq2WhlTrqFrnt/No Transmission ==
  EMTrqCmd : Inport
  EMSpd : Inport  Port=2
  Divide2 : Product  Inputs=**
  Dual EMs : Gain  Gain=2
  Gain3 : Gain  Gain=PlntEMWhlGearRatioFL
  Gear Eta : Subsystem
  WhlMotTrq : Outport  VectorParamsAs1DForOutWhenUnconnected=off
  wires:
  Dual EMs/1 -> Gain3/1, Gear Eta/2(TrqIn)
  Gear Eta/1(eta) -> Divide2/1
  EMTrqCmd/1 -> Dual EMs/1
  EMSpd/1 -> Gear Eta/1(SpdIn)
  Divide2/1 -> WhlMotTrq/1
  Gain3/1 -> Divide2/2

== system EvPowertrainController2EM_r3/Energy Management/Calculate Average EMSpd and Wheel Torque Curves for Front and Rear Axles/3EM Dual Front/EMTrq2WhlTrqFrnt/Transmission ==
  Gear : Inport
  EMTrqCmd : Inport  Port=2
  EMSpd : Inport  Port=3
  Diff Eta : Subsystem
  Divide : Product  Inputs=**
  Divide1 : Product  Inputs=**
  Divide2 : Product  Inputs=**
  Divide3 : Product  Inputs=*/
  Gain : Gain  Gain=PlntDiffrntlRatio
  Gear ratio look up : LookupNDDirect  NumberOfTableDimensions=1  Table=PlntTransGearRatioVect
  Trans Eta : Subsystem
  WhlMotTrq : Outport  VectorParamsAs1DForOutWhenUnconnected=off
  wires:
  Gain/1 -> Divide2/2
  Gear ratio look up/1 -> Divide3/2, Divide/1
  Divide/1 -> Divide1/2
  Gear/1 -> Trans Eta/3(Gear), Gear ratio look up/1
  Trans Eta/1(eta) -> Divide1/1
  Divide1/1 -> Diff Eta/2(TrqIn), Gain/1
  Divide2/1 -> WhlMotTrq/1
  Diff Eta/1(eta) -> Divide2/1
  [Spd] -> Divide3/1
  Divide3/1 -> Diff Eta/1(SpdIn)
  EMTrqCmd/1 -> Divide/2, Trans Eta/1(TrqIn)
  EMSpd/1 -> [Spd], Trans Eta/2(SpdIn)

== system EvPowertrainController2EM_r3/Energy Management/Calculate Average EMSpd and Wheel Torque Curves for Front and Rear Axles/3EM Dual Front/EMTrq2WhlTrqRear/No Transmission ==
  EMTrqCmd : Inport
  EMSpd : Inport  Port=2
  Diff Eta : Subsystem
  Divide2 : Product  Inputs=**
  Gain3 : Gain  Gain=PlntDiffrntl2Ratio
  WhlMotTrq : Outport  VectorParamsAs1DForOutWhenUnconnected=off
  wires:
  Diff Eta/1(eta) -> Divide2/1
  EMTrqCmd/1 -> Gain3/1, Diff Eta/2(TrqIn)
  EMSpd/1 -> Diff Eta/1(SpdIn)
  Divide2/1 -> WhlMotTrq/1
  Gain3/1 -> Divide2/2

== system EvPowertrainController2EM_r3/Energy Management/Calculate Average EMSpd and Wheel Torque Curves for Front and Rear Axles/3EM Dual Front/EMTrq2WhlTrqRear/Transmission ==
  Gear : Inport
  EMTrqCmd : Inport  Port=2
  EMSpd : Inport  Port=3
  Diff Eta : Subsystem
  Divide : Product  Inputs=**
  Divide1 : Product  Inputs=**
  Divide2 : Product  Inputs=**
  Divide3 : Product  Inputs=*/
  Gain : Gain  Gain=PlntDiffrntl2Ratio
  Gear ratio look up : LookupNDDirect  NumberOfTableDimensions=1  Table=PlntTransGearRatioVect
  Trans Eta : Subsystem
  WhlMotTrq : Outport  VectorParamsAs1DForOutWhenUnconnected=off
  wires:
  EMSpd/1 -> Trans Eta/2(SpdIn), [Spd]
  EMTrqCmd/1 -> Trans Eta/1(TrqIn), Divide/2
  Divide3/1 -> Diff Eta/1(SpdIn)
  [Spd] -> Divide3/1
  Diff Eta/1(eta) -> Divide2/1
  Divide2/1 -> WhlMotTrq/1
  Divide1/1 -> Gain/1, Diff Eta/2(TrqIn)
  Trans Eta/1(eta) -> Divide1/1
  Gear/1 -> Gear ratio look up/1, Trans Eta/3(Gear)
  Divide/1 -> Divide1/2
  Gear ratio look up/1 -> Divide/1, Divide3/2
  Gain/1 -> Divide2/2

== system EvPowertrainController2EM_r3/Energy Management/Calculate Average EMSpd and Wheel Torque Curves for Front and Rear Axles/3EM Dual Rear/EMTrq2WhlTrqFrnt/No Transmission ==
  EMTrqCmd : Inport
  EMSpd : Inport  Port=2
  Diff Eta : Subsystem
  Divide2 : Product  Inputs=**
  Gain3 : Gain  Gain=PlntDiffrntlRatio
  WhlMotTrq : Outport  VectorParamsAs1DForOutWhenUnconnected=off
  wires:
  Gain3/1 -> Divide2/2
  Divide2/1 -> WhlMotTrq/1
  EMSpd/1 -> Diff Eta/1(SpdIn)
  EMTrqCmd/1 -> Diff Eta/2(TrqIn), Gain3/1
  Diff Eta/1(eta) -> Divide2/1

== system EvPowertrainController2EM_r3/Energy Management/Calculate Average EMSpd and Wheel Torque Curves for Front and Rear Axles/3EM Dual Rear/EMTrq2WhlTrqFrnt/Transmission ==
  Gear : Inport
  EMTrqCmd : Inport  Port=2
  EMSpd : Inport  Port=3
  Diff Eta : Subsystem
  Divide : Product  Inputs=**
  Divide1 : Product  Inputs=**
  Divide2 : Product  Inputs=**
  Divide3 : Product  Inputs=*/
  Gain : Gain  Gain=PlntDiffrntlRatio
  Gear ratio look up : LookupNDDirect  NumberOfTableDimensions=1  Table=PlntTransGearRatioVect
  Trans Eta : Subsystem
  WhlMotTrq : Outport  VectorParamsAs1DForOutWhenUnconnected=off
  wires:
  EMSpd/1 -> Trans Eta/2(SpdIn), [Spd]
  EMTrqCmd/1 -> Trans Eta/1(TrqIn), Divide/2
  Divide3/1 -> Diff Eta/1(SpdIn)
  [Spd] -> Divide3/1
  Diff Eta/1(eta) -> Divide2/1
  Divide2/1 -> WhlMotTrq/1
  Divide1/1 -> Gain/1, Diff Eta/2(TrqIn)
  Trans Eta/1(eta) -> Divide1/1
  Gear/1 -> Gear ratio look up/1, Trans Eta/3(Gear)
  Divide/1 -> Divide1/2
  Gear ratio look up/1 -> Divide/1, Divide3/2
  Gain/1 -> Divide2/2

== system EvPowertrainController2EM_r3/Energy Management/Calculate Average EMSpd and Wheel Torque Curves for Front and Rear Axles/3EM Dual Rear/EMTrq2WhlTrqRear/No Transmission ==
  EMTrqCmd : Inport
  EMSpd : Inport  Port=2
  Divide2 : Product  Inputs=**
  Dual EMs : Gain  Gain=2
  Gain3 : Gain  Gain=PlntEMWhlGearRatioRL
  Gear Eta : Subsystem
  WhlMotTrq : Outport  VectorParamsAs1DForOutWhenUnconnected=off
  wires:
  Dual EMs/1 -> Gear Eta/2(TrqIn), Gain3/1
  Gain3/1 -> Divide2/2
  Divide2/1 -> WhlMotTrq/1
  EMSpd/1 -> Gear Eta/1(SpdIn)
  EMTrqCmd/1 -> Dual EMs/1
  Gear Eta/1(eta) -> Divide2/1

== system EvPowertrainController2EM_r3/Energy Management/Calculate Average EMSpd and Wheel Torque Curves for Front and Rear Axles/3EM Dual Rear/EMTrq2WhlTrqRear/Transmission ==
  Gear : Inport
  EMTrqCmd : Inport  Port=2
  EMSpd : Inport  Port=3
  Diff Eta : Subsystem
  Divide : Product  Inputs=**
  Divide1 : Product  Inputs=**
  Divide2 : Product  Inputs=**
  Divide3 : Product  Inputs=*/
  Gain : Gain  Gain=PlntDiffrntl2Ratio
  Gear ratio look up : LookupNDDirect  NumberOfTableDimensions=1  Table=PlntTransGearRatioVect
  Trans Eta : Subsystem
  WhlMotTrq : Outport  VectorParamsAs1DForOutWhenUnconnected=off
  wires:
  Gain/1 -> Divide2/2
  Gear ratio look up/1 -> Divide3/2, Divide/1
  Divide/1 -> Divide1/2
  Gear/1 -> Trans Eta/3(Gear), Gear ratio look up/1
  Trans Eta/1(eta) -> Divide1/1
  Divide1/1 -> Diff Eta/2(TrqIn), Gain/1
  Divide2/1 -> WhlMotTrq/1
  Diff Eta/1(eta) -> Divide2/1
  [Spd] -> Divide3/1
  Divide3/1 -> Diff Eta/1(SpdIn)
  EMTrqCmd/1 -> Divide/2, Trans Eta/1(TrqIn)
  EMSpd/1 -> [Spd], Trans Eta/2(SpdIn)

== system EvPowertrainController2EM_r3/Energy Management/Calculate Average EMSpd and Wheel Torque Curves for Front and Rear Axles/4EM/EMTrq2WhlTrqFrnt/No Transmission ==
  EMTrqCmd : Inport
  EMSpd : Inport  Port=2
  Divide2 : Product  Inputs=**
  Dual EMs : Gain  Gain=2
  Gain3 : Gain  Gain=PlntEMWhlGearRatioFL
  Gear Eta : Subsystem
  WhlMotTrq : Outport  VectorParamsAs1DForOutWhenUnconnected=off
  wires:
  Dual EMs/1 -> Gain3/1, Gear Eta/2(TrqIn)
  Gear Eta/1(eta) -> Divide2/1
  EMTrqCmd/1 -> Dual EMs/1
  EMSpd/1 -> Gear Eta/1(SpdIn)
  Divide2/1 -> WhlMotTrq/1
  Gain3/1 -> Divide2/2

== system EvPowertrainController2EM_r3/Energy Management/Calculate Average EMSpd and Wheel Torque Curves for Front and Rear Axles/4EM/EMTrq2WhlTrqFrnt/Transmission ==
  Gear : Inport
  EMTrqCmd : Inport  Port=2
  EMSpd : Inport  Port=3
  Diff Eta : Subsystem
  Divide : Product  Inputs=**
  Divide1 : Product  Inputs=**
  Divide2 : Product  Inputs=**
  Divide3 : Product  Inputs=*/
  Gain : Gain  Gain=PlntDiffrntlRatio
  Gear ratio look up : LookupNDDirect  NumberOfTableDimensions=1  Table=PlntTransGearRatioVect
  Trans Eta : Subsystem
  WhlMotTrq : Outport  VectorParamsAs1DForOutWhenUnconnected=off
  wires:
  Gain/1 -> Divide2/2
  Gear ratio look up/1 -> Divide3/2, Divide/1
  Divide/1 -> Divide1/2
  Gear/1 -> Trans Eta/3(Gear), Gear ratio look up/1
  Trans Eta/1(eta) -> Divide1/1
  Divide1/1 -> Diff Eta/2(TrqIn), Gain/1
  Divide2/1 -> WhlMotTrq/1
  Diff Eta/1(eta) -> Divide2/1
  [Spd] -> Divide3/1
  Divide3/1 -> Diff Eta/1(SpdIn)
  EMTrqCmd/1 -> Divide/2, Trans Eta/1(TrqIn)
  EMSpd/1 -> [Spd], Trans Eta/2(SpdIn)

== system EvPowertrainController2EM_r3/Energy Management/Calculate Average EMSpd and Wheel Torque Curves for Front and Rear Axles/4EM/EMTrq2WhlTrqRear/No Transmission ==
  EMTrqCmd : Inport
  EMSpd : Inport  Port=2
  Divide2 : Product  Inputs=**
  Dual EMs : Gain  Gain=2
  Gain3 : Gain  Gain=PlntEMWhlGearRatioRL
  Gear Eta : Subsystem
  WhlMotTrq : Outport  VectorParamsAs1DForOutWhenUnconnected=off
  wires:
  Dual EMs/1 -> Gain3/1, Gear Eta/2(TrqIn)
  Gear Eta/1(eta) -> Divide2/1
  EMTrqCmd/1 -> Dual EMs/1
  EMSpd/1 -> Gear Eta/1(SpdIn)
  Divide2/1 -> WhlMotTrq/1
  Gain3/1 -> Divide2/2
